simulink library "Hquad_control_LIB_LQR"  (Simulink 7.6)
settings: Solver=ode45  StartTime=0.0  StopTime=10.0  RelTol=1e-3
values from neighbouring files (symbols this model uses):
  g = 9.8065    [kostas_malakies.mat]    (also in kostas_malakies2.mat; load_PMModel.m = 9.81; main.m; main_last.m)
  K_lqr_x = [-0.863276621575 -0.709547355686 0.590253339062]    [kostas_malakies.mat]    (also in kostas_malakies2.mat)
  K_lqr_y = [0.862865129123 0.706975959941 0.571517383363]    [kostas_malakies.mat]    (also in kostas_malakies2.mat)
  K_lqr_yaw = [2.45277664624 0.892670523904]    [kostas_malakies.mat]    (also in kostas_malakies2.mat)
  K_lqr_z = [-2.51059156801 -2.42233318314]    [kostas_malakies.mat]    (also in kostas_malakies2.mat)
  mass = 0.66    [kostas_malakies.mat]    (also in kostas_malakies2.mat; load_PMModel.m = 0.687; main_last.m)
  MAX_ANGLE = 0.261799387799    [kostas_malakies.mat]    (also in kostas_malakies2.mat; main.m; main_last.m)
  MAX_FORCE = 2    [kostas_malakies.mat]    (also in kostas_malakies2.mat; main.m; main_last.m)
  MAX_YAW_RATE = 3.14159265359    [kostas_malakies.mat]    (also in kostas_malakies2.mat; main.m; main_last.m)
  traj_FG =     [kostas.mat]    (also in kostas_malakies.mat; kostas_malakies2.mat; main_last.m = ReferenceCreator(maxdisty,maxdistz,scale_y,scale_z); traj_helix.mat)
libraries: Hquad_control_LIB_LQR x13, simulink x9, Hquad_control_LIB_MPC x8
settings Model: Creator=andi  LastModifiedBy=burrimi

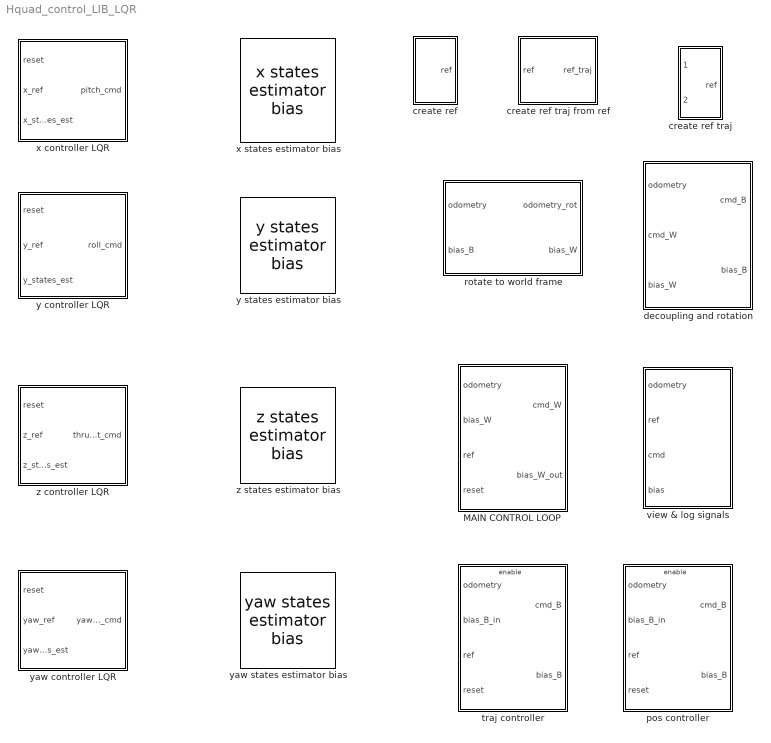
== system Hquad_control_LIB_LQR ==
  MAIN CONTROL LOOP : Subsystem  Priority=2  TreatAsAtomicUnit=on
  create ref : Subsystem
  create ref traj : Subsystem
  create ref traj from ref : Subsystem
  decoupling and rotation : Subsystem  Priority=3  TreatAsAtomicUnit=on
  pos controller : Subsystem
  rotate to world frame : Subsystem  Priority=1
  traj controller : Subsystem
  view & log signals : Subsystem
  "x controller LQR  " : Subsystem
  x states estimator bias : Hquad_control_LIB_MPC/x states estimator bias  SystemSampleTime=-1
  y controller LQR : Subsystem
  y states estimator bias : Hquad_control_LIB_MPC/y states estimator bias  SystemSampleTime=-1
  yaw controller LQR : Subsystem
  yaw states estimator bias : Hquad_control_LIB_MPC/yaw states estimator bias  SystemSampleTime=-1
  z controller LQR : Subsystem
  z states estimator bias : Hquad_control_LIB_MPC/z states estimator bias  SystemSampleTime=-1

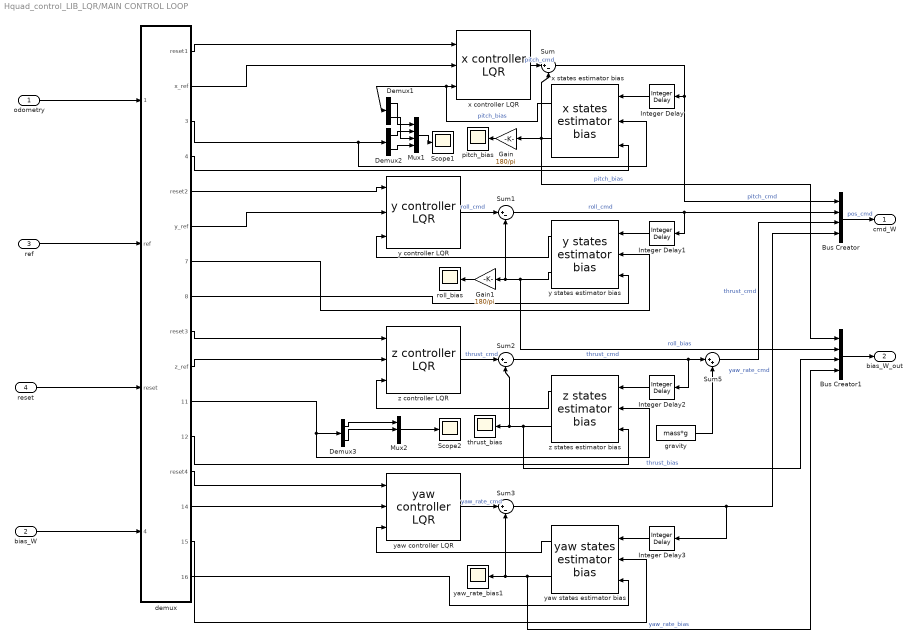
== system Hquad_control_LIB_LQR/MAIN CONTROL LOOP ==
  odometry : Inport
  bias_W : Inport  Port=2
  ref : Inport  Port=3
  reset : Inport  Port=4
  Bus Creator : BusCreator
  Bus Creator1 : BusCreator
  Demux1 : Demux  Outputs=3
  Demux2 : Demux  Outputs=3
  Demux3 : Demux  Outputs=2
  Gain : Gain  Gain=180/pi
  Gain1 : Gain  Gain=180/pi
  Integer Delay{,1..3} (4 alike) : simulink/Discrete/Integer Delay  NumDelays=1  vinit=0.0  samptime=-1
  Mux1 : Mux
  Mux2 : Mux  Inputs=5
  Scope1 : Scope
      settings: YMin=-0.05  YMax=1.05  SaveName=ScopeData6
  Scope2 : Scope
      settings: YMin=-0.4  YMax=1.4  SaveName=ScopeData15
  Sum{,1..3} (4 alike) : Sum  Inputs=|+-
  Sum5 : Sum  Inputs=|++
  demux : Subsystem
  gravity : Constant  Value=mass*g
  pitch_bias : Scope
      settings: YMin=0  YMax=3.75  SaveName=ScopeData7
  roll_bias : Scope
      settings: YMin=-1  YMax=1  SaveName=ScopeData12
  thrust_bias : Scope
      settings: YMin=0  YMax=0.3  SaveName=ScopeData13
  "x controller LQR  " : Hquad_control_LIB_LQR/x controller LQR    SystemSampleTime=-1
  x states estimator bias : Hquad_control_LIB_MPC/x states estimator bias  SystemSampleTime=-1
  y controller LQR : Hquad_control_LIB_LQR/y controller LQR  SystemSampleTime=-1
  y states estimator bias : Hquad_control_LIB_MPC/y states estimator bias  SystemSampleTime=-1
  yaw controller LQR : Hquad_control_LIB_LQR/yaw controller LQR  SystemSampleTime=-1
  yaw states estimator bias : Hquad_control_LIB_MPC/yaw states estimator bias  SystemSampleTime=-1
  yaw_rate_bias1 : Scope
      settings: YMin=-1  YMax=1  SaveName=ScopeData16
  z controller LQR : Hquad_control_LIB_LQR/z controller LQR  SystemSampleTime=-1
  z states estimator bias : Hquad_control_LIB_MPC/z states estimator bias  SystemSampleTime=-1
  cmd_W : Outport
  bias_W_out : Outport  Port=2
  wires:
  x states estimator bias/1 -> Demux1/1, "x controller LQR  "/3  "pitch_bias"
  demux/14(yaw_ref) -> yaw controller LQR/2
  demux/11(z_states_meas) -> Demux3/1, z states estimator bias/2
  demux/7(y_states_meas) -> y states estimator bias/2
  demux/3(x_states_meas) -> Demux2/1, x states estimator bias/2
  Bus Creator/1 -> cmd_W/1  "pos_cmd"
  demux/13(reset4) -> yaw controller LQR/1
  demux/9(reset3) -> z controller LQR/1
  demux/6(y_ref) -> y controller LQR/2
  demux/5(reset2) -> y controller LQR/1
  demux/1(reset1) -> "x controller LQR  "/1
  reset/1 -> demux/3(reset)
  ref/1 -> demux/2(ref)
  odometry/1 -> demux/1(odometry)
  Integer Delay2/1 -> z states estimator bias/1
  Integer Delay1/1 -> y states estimator bias/1
  demux/2(x_ref) -> "x controller LQR  "/2
  demux/10(z_ref) -> z controller LQR/2
  z states estimator bias/1 -> z controller LQR/3
  Mux2/1 -> Scope2/1
  Demux3/1 -> Mux2/1
  Demux3/2 -> Mux2/3
  Integer Delay/1 -> x states estimator bias/1
  y states estimator bias/1 -> y controller LQR/3
  Demux1/1 -> Mux1/1
  Demux2/1 -> Mux1/2
  Mux1/1 -> Scope1/1
  "x controller LQR  "/1 -> Sum/1  "pitch_cmd"
  Sum/1 -> Integer Delay/1, Bus Creator/1  "pitch_cmd"
  y controller LQR/1 -> Sum1/1  "roll_cmd"
  Sum1/1 -> Integer Delay1/1, Bus Creator/2  "roll_cmd"
  y states estimator bias/2 -> Gain1/1, Sum1/2, Bus Creator1/2  "roll_bias"
  z states estimator bias/2 -> Bus Creator1/3, thrust_bias/1, Sum2/2  "thrust_bias"
  z controller LQR/1 -> Sum2/1  "thrust_cmd"
  Sum2/1 -> Integer Delay2/1, Sum5/1  "thrust_cmd"
  Bus Creator1/1 -> bias_W_out/1
  gravity/1 -> Sum5/2
  Sum5/1 -> Bus Creator/3  "thrust_cmd"
  Gain/1 -> pitch_bias/1
  Gain1/1 -> roll_bias/1
  demux/15(yaw_states_meas) -> yaw states estimator bias/2
  Demux1/3 -> Mux1/3
  Demux2/3 -> Mux1/4
  x states estimator bias/2 -> Gain/1, Bus Creator1/1, Sum/2  "pitch_bias"
  Integer Delay3/1 -> yaw states estimator bias/1
  yaw states estimator bias/1 -> yaw controller LQR/3
  yaw states estimator bias/2 -> yaw_rate_bias1/1, Sum3/2, Bus Creator1/4  "yaw_rate_bias"
  yaw controller LQR/1 -> Sum3/1  "yaw_rate_cmd"
  Sum3/1 -> Bus Creator/4, Integer Delay3/1  "yaw_rate_cmd"
  bias_W/1 -> demux/4(bias_W)
  demux/16(yaw_rate_bias) -> yaw states estimator bias/3
  demux/12(thrust_bias) -> z states estimator bias/3
  demux/8(roll_bias) -> y states estimator bias/3
  demux/4(pitch_bias) -> x states estimator bias/3

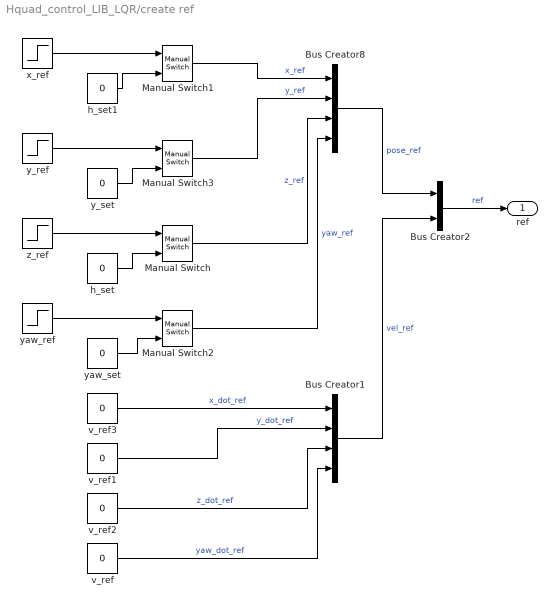
== system Hquad_control_LIB_LQR/create ref ==
  Bus Creator1 : BusCreator
  Bus Creator2 : BusCreator  Inputs=2
  Bus Creator8 : BusCreator
  Manual Switch{,1..3} (4 alike) : simulink/Signal Routing/Manual Switch  SystemSampleTime=-1  sw=1  action=0  varsize=off
  h_set : Constant  Value=0  OutDataTypeStr=double  SampleTime=-1
  h_set1 : Constant  Value=0  OutDataTypeStr=double  SampleTime=-1
  v_ref{,1..3} (4 alike) : Constant  Value=0  OutDataTypeStr=double  SampleTime=-1
  x_ref : Step  Time=5  SampleTime=0
  y_ref : Step  Time=15  SampleTime=0
  y_set : Constant  Value=0  OutDataTypeStr=double  SampleTime=-1
  yaw_ref : Step  Time=20  After=pi  SampleTime=0
  "yaw_set  " : Constant  Value=0  OutDataTypeStr=double  SampleTime=-1
  z_ref : Step  Time=15  SampleTime=0
  ref : Outport
  wires:
  yaw_ref/1 -> Manual Switch2/1
  "yaw_set  "/1 -> Manual Switch2/2
  h_set/1 -> Manual Switch/2
  z_ref/1 -> Manual Switch/1
  y_ref/1 -> Manual Switch3/1
  y_set/1 -> Manual Switch3/2
  h_set1/1 -> Manual Switch1/2
  Bus Creator2/1 -> ref/1  "ref"
  Bus Creator8/1 -> Bus Creator2/1  "pose_ref"
  Bus Creator1/1 -> Bus Creator2/2  "vel_ref"
  Manual Switch1/1 -> Bus Creator8/1  "x_ref"
  Manual Switch3/1 -> Bus Creator8/2  "y_ref"
  Manual Switch2/1 -> Bus Creator8/4  "yaw_ref"
  Manual Switch/1 -> Bus Creator8/3  "z_ref"
  v_ref/1 -> Bus Creator1/4  "yaw_dot_ref"
  v_ref3/1 -> Bus Creator1/1  "x_dot_ref"
  v_ref1/1 -> Bus Creator1/2  "y_dot_ref"
  v_ref2/1 -> Bus Creator1/3  "z_dot_ref"
  x_ref/1 -> Manual Switch1/1

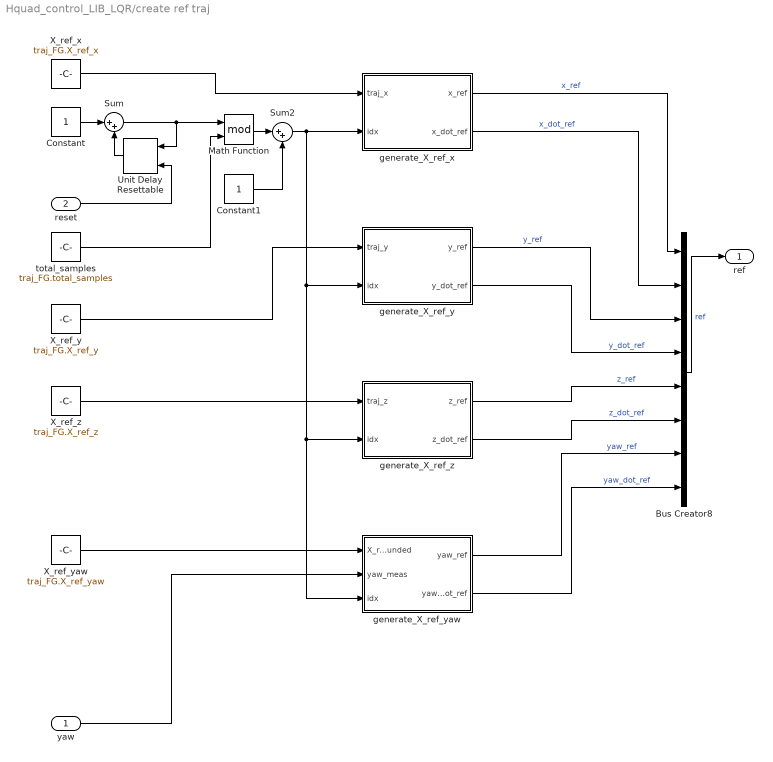
== system Hquad_control_LIB_LQR/create ref traj ==
  yaw : Inport
  reset : Inport  Port=2
  Bus Creator8 : BusCreator  Inputs=8
  Constant : Constant
  Constant1 : Constant
  Math Function : Math  Operator=mod  SaturateOnIntegerOverflow=on
  Sum : Sum  Inputs=|++
  Sum2 : Sum  Inputs=|++
  Unit Delay Resettable : simulink/Additional Math & Discrete/Additional Discrete/Unit Delay Resettable  SystemSampleTime=-1  vinit=0.0  tsamp=-1
  X_ref_x : Constant  Value=traj_FG.X_ref_x
  X_ref_y : Constant  Value=traj_FG.X_ref_y
  X_ref_yaw : Constant  Value=traj_FG.X_ref_yaw
  X_ref_z : Constant  Value=traj_FG.X_ref_z
  generate_X_ref_x : Stateflow chart  TreatAsAtomicUnit=on
  generate_X_ref_y : Stateflow chart  TreatAsAtomicUnit=on
  generate_X_ref_yaw : Stateflow chart  TreatAsAtomicUnit=on
  generate_X_ref_z : Stateflow chart  TreatAsAtomicUnit=on
  total_samples : Constant  Value=traj_FG.total_samples
  ref : Outport
  wires:
  reset/1 -> Unit Delay Resettable/2
  Bus Creator8/1 -> ref/1  "ref"
  Constant/1 -> Sum/1
  Unit Delay Resettable/1 -> Sum/2
  Sum/1 -> Unit Delay Resettable/1, Math Function/1
  total_samples/1 -> Math Function/2
  Math Function/1 -> Sum2/1
  X_ref_yaw/1 -> generate_X_ref_yaw/1(X_ref_yaw_unbounded)
  Constant1/1 -> Sum2/2
  yaw/1 -> generate_X_ref_yaw/2(yaw_meas)
  Sum2/1 -> generate_X_ref_x/2(idx), generate_X_ref_yaw/3(idx), generate_X_ref_z/2(idx), generate_X_ref_y/2(idx)
  X_ref_z/1 -> generate_X_ref_z/1(traj_z)
  X_ref_y/1 -> generate_X_ref_y/1(traj_y)
  X_ref_x/1 -> generate_X_ref_x/1(traj_x)
  generate_X_ref_yaw/2(yaw_dot_ref) -> Bus Creator8/8  "yaw_dot_ref"
  generate_X_ref_yaw/1(yaw_ref) -> Bus Creator8/7  "yaw_ref"
  generate_X_ref_z/2(z_dot_ref) -> Bus Creator8/6  "z_dot_ref"
  generate_X_ref_z/1(z_ref) -> Bus Creator8/5  "z_ref"
  generate_X_ref_y/2(y_dot_ref) -> Bus Creator8/4  "y_dot_ref"
  generate_X_ref_y/1(y_ref) -> Bus Creator8/3  "y_ref"
  generate_X_ref_x/2(x_dot_ref) -> Bus Creator8/2  "x_dot_ref"
  generate_X_ref_x/1(x_ref) -> Bus Creator8/1  "x_ref"

== system Hquad_control_LIB_LQR/create ref traj from ref ==
  ref : Inport
  Bus Creator8 : BusCreator
  Bus Selector1 : BusSelector  OutputSignals=pose_ref.x_ref,vel_ref.x_dot_ref,pose_ref.y_ref,vel_ref.y_dot_ref,pose_ref.z_ref,vel_ref.z_dot_ref,pose_ref.yaw_ref,vel_ref.yaw_dot_ref
  generate_X_ref_x : Stateflow chart  TreatAsAtomicUnit=on
  generate_X_ref_y : Stateflow chart  TreatAsAtomicUnit=on
  generate_X_ref_yaw : Stateflow chart  TreatAsAtomicUnit=on
  generate_X_ref_z : Stateflow chart  TreatAsAtomicUnit=on
  ref_traj : Outport
  wires:
  Bus Creator8/1 -> ref_traj/1  "ref"
  generate_X_ref_x/1(X_ref) -> Bus Creator8/1  "X_ref_x"
  generate_X_ref_y/1(X_ref) -> Bus Creator8/2  "X_ref_y"
  generate_X_ref_z/1(X_ref) -> Bus Creator8/3  "X_ref_z"
  generate_X_ref_yaw/1(X_ref) -> Bus Creator8/4  "X_ref_yaw"
  ref/1 -> Bus Selector1/1
  Bus Selector1/1 -> generate_X_ref_x/1(x_ref)  "<x_ref>"
  Bus Selector1/2 -> generate_X_ref_x/2(x_dot_ref)  "<x_dot_ref>"
  Bus Selector1/3 -> generate_X_ref_y/1(x_ref)  "<y_ref>"
  Bus Selector1/4 -> generate_X_ref_y/2(x_dot_ref)  "<y_dot_ref>"
  Bus Selector1/5 -> generate_X_ref_z/1(x_ref)  "<z_ref>"
  Bus Selector1/6 -> generate_X_ref_z/2(x_dot_ref)  "<z_dot_ref>"
  Bus Selector1/7 -> generate_X_ref_yaw/1(x_ref)  "<yaw_ref>"
  Bus Selector1/8 -> generate_X_ref_yaw/2(x_dot_ref)  "<yaw_dot_ref>"

== system Hquad_control_LIB_LQR/decoupling and rotation ==
  note: 
  odometry : Inport
  cmd_W : Inport  Port=2
  bias_W : Inport  Port=3
  Bus Selector1 : BusSelector  OutputSignals=rpy.yaw
  Bus Selector2 : BusSelector  OutputSignals=rpy.roll,rpy.pitch
  "decoupling " : Subsystem
  rotate_to_quat_frame : Subsystem
  cmd_B : Outport
  bias_B : Outport  Port=2
  wires:
  rotate_to_quat_frame/1("cmd_rot  ") -> cmd_B/1  "roll_cmd"
  "decoupling "/1("cmd_comp  ") -> rotate_to_quat_frame/2(cmd_comp)  "thrust_cmd"
  odometry/1 -> Bus Selector1/1, Bus Selector2/1
  Bus Selector1/1 -> rotate_to_quat_frame/1(yaw_meas)  "<yaw>"
  rotate_to_quat_frame/2(bias_rot) -> bias_B/1
  bias_W/1 -> rotate_to_quat_frame/3(bias)
  cmd_W/1 -> "decoupling "/3(cmd)
  Bus Selector2/1 -> "decoupling "/1("roll_meas  ")  "<roll>"
  Bus Selector2/2 -> "decoupling "/2("pitch_meas  ")  "<pitch>"

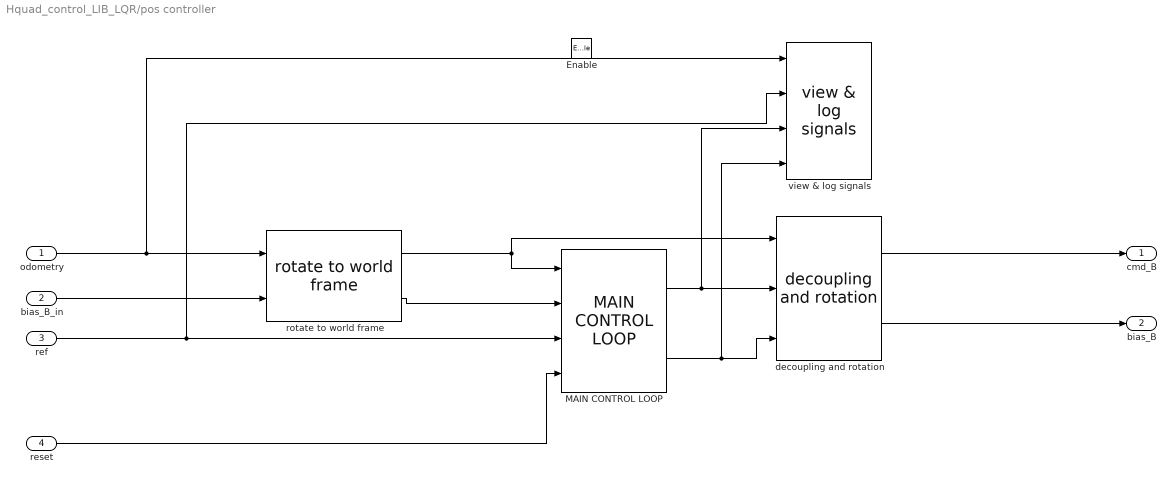
== system Hquad_control_LIB_LQR/pos controller ==
  odometry : Inport
  bias_B_in : Inport  Port=2
  ref : Inport  Port=3
  reset : Inport  Port=4
  Enable : EnablePort  StatesWhenEnabling=reset
  MAIN CONTROL LOOP : Hquad_control_LIB_LQR/MAIN CONTROL LOOP  Priority=2  SystemSampleTime=-1
  decoupling and rotation : Hquad_control_LIB_LQR/decoupling and rotation  Priority=3  SystemSampleTime=-1
  rotate to world frame : Hquad_control_LIB_LQR/rotate to world frame  Priority=1  SystemSampleTime=-1
  view & log signals : Hquad_control_LIB_LQR/view & log signals  SystemSampleTime=-1
  cmd_B : Outport
  bias_B : Outport  Port=2
  wires:
  MAIN CONTROL LOOP/1 -> view & log signals/3, decoupling and rotation/2
  odometry/1 -> view & log signals/1, rotate to world frame/1
  reset/1 -> MAIN CONTROL LOOP/4
  ref/1 -> view & log signals/2, MAIN CONTROL LOOP/3
  rotate to world frame/1 -> decoupling and rotation/1, MAIN CONTROL LOOP/1
  MAIN CONTROL LOOP/2 -> view & log signals/4, decoupling and rotation/3
  decoupling and rotation/1 -> cmd_B/1
  decoupling and rotation/2 -> bias_B/1
  rotate to world frame/2 -> MAIN CONTROL LOOP/2
  bias_B_in/1 -> rotate to world frame/2

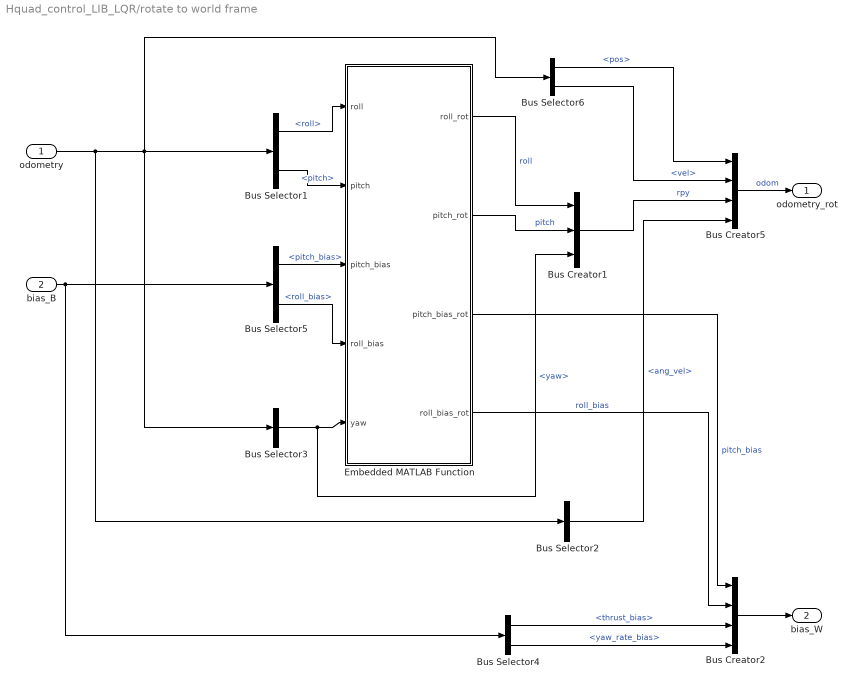
== system Hquad_control_LIB_LQR/rotate to world frame ==
  odometry : Inport
  bias_B : Inport  Port=2
  Bus Creator1 : BusCreator  Inputs=3
  Bus Creator2 : BusCreator
  Bus Creator5 : BusCreator
  Bus Selector1 : BusSelector  OutputSignals=rpy.roll,rpy.pitch
  Bus Selector2 : BusSelector  OutputSignals=ang_vel
  Bus Selector3 : BusSelector  OutputSignals=rpy.yaw
  Bus Selector4 : BusSelector  OutputSignals=thrust_bias,yaw_rate_bias
  Bus Selector5 : BusSelector  OutputSignals=pitch_bias,roll_bias
  Bus Selector6 : BusSelector  OutputSignals=pos,vel
  Embedded MATLAB Function : Stateflow chart  TreatAsAtomicUnit=on
  odometry_rot : Outport
  bias_W : Outport  Port=2
  wires:
  Bus Selector6/2 -> Bus Creator5/2  "<vel>"
  Bus Selector6/1 -> Bus Creator5/1  "<pos>"
  Bus Creator5/1 -> odometry_rot/1  "odom"
  Bus Selector3/1 -> Embedded MATLAB Function/5(yaw), Bus Creator1/3  "<yaw>"
  odometry/1 -> Bus Selector3/1, Bus Selector1/1, Bus Selector6/1, Bus Selector2/1
  Bus Selector2/1 -> Bus Creator5/4  "<ang_vel>"
  Bus Creator1/1 -> Bus Creator5/3  "rpy"
  Embedded MATLAB Function/1(roll_rot) -> Bus Creator1/1  "roll"
  Embedded MATLAB Function/2(pitch_rot) -> Bus Creator1/2  "pitch"
  Bus Selector1/1 -> Embedded MATLAB Function/1(roll)  "<roll>"
  Bus Selector1/2 -> Embedded MATLAB Function/2(pitch)  "<pitch>"
  Bus Creator2/1 -> bias_W/1
  Bus Selector4/2 -> Bus Creator2/4  "<yaw_rate_bias>"
  Bus Selector4/1 -> Bus Creator2/3  "<thrust_bias>"
  Bus Selector5/1 -> Embedded MATLAB Function/3(pitch_bias)  "<pitch_bias>"
  Bus Selector5/2 -> Embedded MATLAB Function/4(roll_bias)  "<roll_bias>"
  bias_B/1 -> Bus Selector5/1, Bus Selector4/1
  Embedded MATLAB Function/3(pitch_bias_rot) -> Bus Creator2/1  "pitch_bias"
  Embedded MATLAB Function/4(roll_bias_rot) -> Bus Creator2/2  "roll_bias"

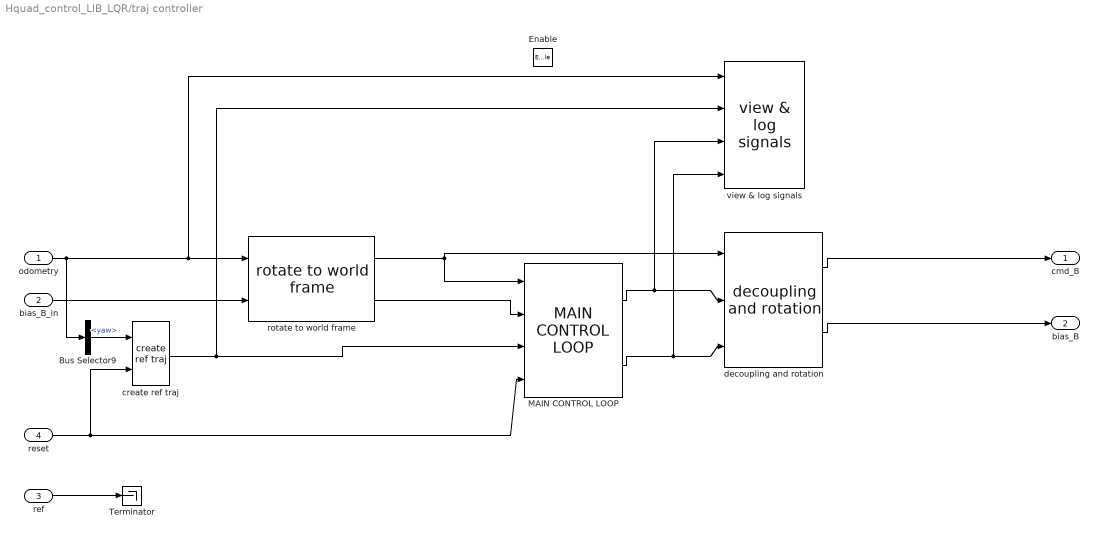
== system Hquad_control_LIB_LQR/traj controller ==
  odometry : Inport
  bias_B_in : Inport  Port=2
  ref : Inport  Port=3
  reset : Inport  Port=4
  Enable : EnablePort  StatesWhenEnabling=reset
  Bus Selector9 : BusSelector  OutputSignals=rpy.yaw
  MAIN CONTROL LOOP : Hquad_control_LIB_LQR/MAIN CONTROL LOOP  Priority=2  SystemSampleTime=-1
  Terminator : Terminator
  create ref traj : Hquad_control_LIB_LQR/create ref traj  SystemSampleTime=-1
  decoupling and rotation : Hquad_control_LIB_LQR/decoupling and rotation  Priority=3  SystemSampleTime=-1
  rotate to world frame : Hquad_control_LIB_LQR/rotate to world frame  Priority=1  SystemSampleTime=-1
  view & log signals : Hquad_control_LIB_LQR/view & log signals  SystemSampleTime=-1
  cmd_B : Outport
  bias_B : Outport  Port=2
  wires:
  ref/1 -> Terminator/1
  Bus Selector9/1 -> create ref traj/1  "<yaw>"
  bias_B_in/1 -> rotate to world frame/2
  rotate to world frame/2 -> MAIN CONTROL LOOP/2
  decoupling and rotation/2 -> bias_B/1
  decoupling and rotation/1 -> cmd_B/1
  MAIN CONTROL LOOP/2 -> decoupling and rotation/3, view & log signals/4
  reset/1 -> create ref traj/2, MAIN CONTROL LOOP/4
  odometry/1 -> Bus Selector9/1, rotate to world frame/1, view & log signals/1
  MAIN CONTROL LOOP/1 -> decoupling and rotation/2, view & log signals/3
  rotate to world frame/1 -> MAIN CONTROL LOOP/1, decoupling and rotation/1
  create ref traj/1 -> MAIN CONTROL LOOP/3, view & log signals/2

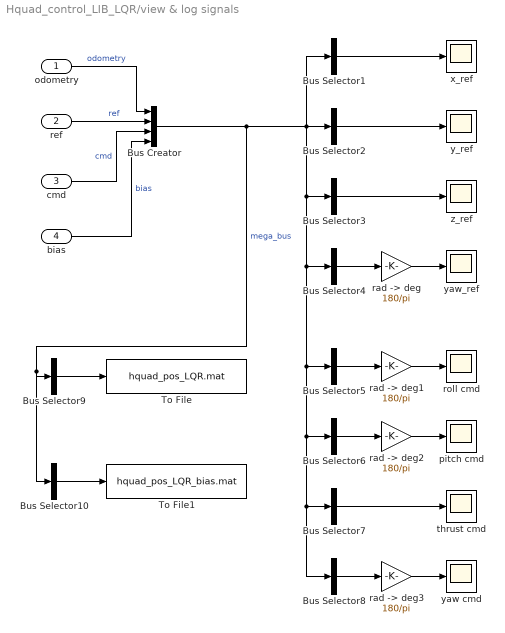
== system Hquad_control_LIB_LQR/view & log signals ==
  odometry : Inport
  ref : Inport  Port=2
  cmd : Inport  Port=3
  bias : Inport  Port=4
  Bus Creator : BusCreator
  Bus Selector1 : BusSelector  OutputSignals=odometry.pos.x,odometry.vel.x_dot,ref.pose_ref.x_ref,ref.vel_ref.x_dot_ref  OutputAsBus=on
  Bus Selector10 : BusSelector  OutputSignals=bias.pitch_bias,bias.roll_bias,bias.thrust_bias,bias.yaw_rate_bias  OutputAsBus=on
  Bus Selector2 : BusSelector  OutputSignals=odometry.pos.y,odometry.vel.y_dot,ref.pose_ref.y_ref,ref.vel_ref.y_dot_ref  OutputAsBus=on
  Bus Selector3 : BusSelector  OutputSignals=odometry.pos.z,odometry.vel.z_dot,ref.pose_ref.z_ref,ref.vel_ref.z_dot_ref  OutputAsBus=on
  Bus Selector4 : BusSelector  OutputSignals=odometry.rpy.yaw,odometry.ang_vel.ang_vel_z,ref.pose_ref.yaw_ref,ref.vel_ref.yaw_dot_ref  OutputAsBus=on
  Bus Selector5 : BusSelector  OutputSignals=odometry.rpy.roll,odometry.ang_vel.ang_vel_x,cmd.roll_cmd  OutputAsBus=on
  Bus Selector6 : BusSelector  OutputSignals=odometry.rpy.pitch,odometry.ang_vel.ang_vel_y,cmd.pitch_cmd  OutputAsBus=on
  Bus Selector7 : BusSelector  OutputSignals=odometry.pos.z,ref.pose_ref.z_ref,cmd.thrust_cmd  OutputAsBus=on
  Bus Selector8 : BusSelector  OutputSignals=odometry.rpy.yaw,odometry.ang_vel.ang_vel_z,cmd.yaw_rate_cmd  OutputAsBus=on
  Bus Selector9 : BusSelector  OutputSignals=odometry.pos.x,odometry.vel.x_dot,odometry.rpy.pitch,ref.pose_ref.x_ref,cmd.pitch_cmd,odometry.pos.y,odometry.vel.y_dot,odometry.rpy.roll,ref.pose_ref.y_ref,cmd.roll_cmd,odometry.pos.z,odometry.vel.z_dot,ref.pose_ref.z_ref,cmd.thrust_cmd,odometry.rpy.yaw,odometry.ang_vel.ang_vel_z,ref.pose_ref.yaw_ref,cmd.yaw_rate_cmd  OutputAsBus=on
  To File : ToFile  Filename=hquad_pos_LQR.mat  MatrixName=hquad_pos_LQR
  To File1 : ToFile  Filename=hquad_pos_LQR_bias.mat  MatrixName=hquad_pos_LQR_bias
  pitch cmd : Scope
      settings: YMin=-15  YMax=15  SaveName=ScopeData2
  rad -> deg{,1..3} (4 alike) : Gain  Gain=180/pi
  roll cmd : Scope
      settings: YMin=-100  YMax=100
  thrust cmd : Scope
      settings: YMin=-3  YMax=3  SaveName=ScopeData11
  x_ref : Scope
      settings: TimeRange=40  YMin=-1.5  YMax=1.5  SaveName=ScopeData3
  y_ref : Scope
      settings: TimeRange=40  YMin=-0.75  YMax=2.75
  yaw cmd : Scope
      settings: YMin=-60  YMax=-0  SaveName=ScopeData10
  yaw_ref : Scope
      settings: TimeRange=39.996  YMin=-1.5  YMax=8.5  SaveName=ScopeData8
  z_ref : Scope
      settings: TimeRange=40  YMin=-21  YMax=1  SaveName=ScopeData5
  wires:
  Bus Selector9/1 -> To File/1
  "rad -> deg"/1 -> yaw_ref/1
  "rad -> deg1"/1 -> roll cmd/1
  "rad -> deg2"/1 -> pitch cmd/1
  "rad -> deg3"/1 -> yaw cmd/1
  odometry/1 -> Bus Creator/1  "odometry"
  ref/1 -> Bus Creator/2  "ref"
  cmd/1 -> Bus Creator/3  "cmd"
  Bus Creator/1 -> Bus Selector1/1, Bus Selector2/1, Bus Selector3/1, Bus Selector4/1, Bus Selector5/1, Bus Selector6/1, Bus Selector7/1, Bus Selector8/1, Bus Selector9/1, Bus Selector10/1  "mega_bus"
  Bus Selector1/1 -> x_ref/1
  Bus Selector2/1 -> y_ref/1
  Bus Selector3/1 -> z_ref/1
  Bus Selector4/1 -> "rad -> deg"/1
  Bus Selector7/1 -> thrust cmd/1
  Bus Selector5/1 -> "rad -> deg1"/1
  Bus Selector6/1 -> "rad -> deg2"/1
  Bus Selector8/1 -> "rad -> deg3"/1
  bias/1 -> Bus Creator/4  "bias"
  Bus Selector10/1 -> To File1/1

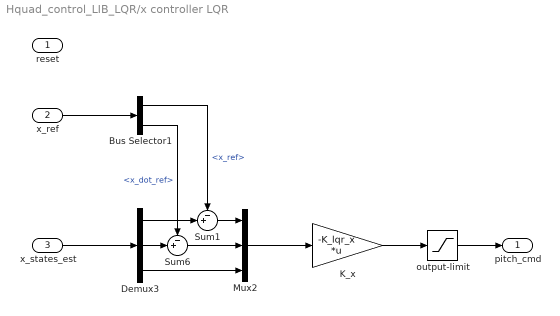
== system Hquad_control_LIB_LQR/x controller LQR   ==
  reset : Inport  PortDimensions=1
  "x_ref  " : Inport  Port=2  PortDimensions=2
  "x_states_est  " : Inport  Port=3
  Bus Selector1 : BusSelector  OutputSignals=x_ref,x_dot_ref
  Demux3 : Demux  Outputs=3
  K_x : Gain  Gain=-K_lqr_x  Multiplication=Matrix(K*u)
  Mux2 : Mux  Inputs=3
  Sum1 : Sum  Inputs=-+|
  Sum6 : Sum  Inputs=-+|
  output-limit : Saturate  UpperLimit=MAX_ANGLE  LowerLimit=-MAX_ANGLE
  "pitch_cmd   " : Outport  PortDimensions=1
  wires:
  Demux3/3 -> Mux2/3
  Demux3/2 -> Sum6/2
  Bus Selector1/2 -> Sum6/1  "<x_dot_ref>"
  Bus Selector1/1 -> Sum1/1  "<x_ref>"
  Sum6/1 -> Mux2/2
  "x_ref  "/1 -> Bus Selector1/1
  K_x/1 -> output-limit/1
  output-limit/1 -> "pitch_cmd   "/1
  "x_states_est  "/1 -> Demux3/1
  Mux2/1 -> K_x/1
  Demux3/1 -> Sum1/2
  Sum1/1 -> Mux2/1

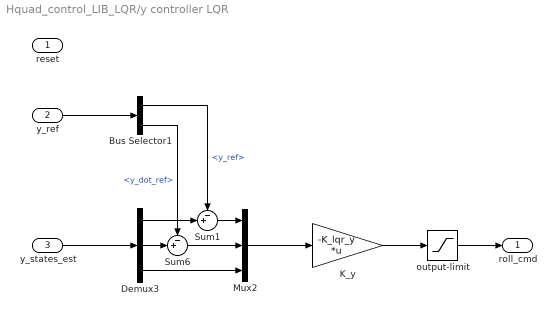
== system Hquad_control_LIB_LQR/y controller LQR ==
  reset : Inport  PortDimensions=1
  "y_ref " : Inport  Port=2  PortDimensions=2
  y_states_est : Inport  Port=3
  Bus Selector1 : BusSelector  OutputSignals=y_ref,y_dot_ref
  Demux3 : Demux  Outputs=3
  K_y : Gain  Gain=-K_lqr_y  Multiplication=Matrix(K*u)
  Mux2 : Mux  Inputs=3
  Sum1 : Sum  Inputs=-+|
  Sum6 : Sum  Inputs=-+|
  output-limit : Saturate  UpperLimit=MAX_ANGLE  LowerLimit=-MAX_ANGLE
  "roll_cmd   " : Outport  PortDimensions=1
  wires:
  Demux3/3 -> Mux2/3
  Demux3/2 -> Sum6/2
  Bus Selector1/2 -> Sum6/1  "<y_dot_ref>"
  Bus Selector1/1 -> Sum1/1  "<y_ref>"
  Sum6/1 -> Mux2/2
  "y_ref "/1 -> Bus Selector1/1
  K_y/1 -> output-limit/1
  output-limit/1 -> "roll_cmd   "/1
  y_states_est/1 -> Demux3/1
  Mux2/1 -> K_y/1
  Demux3/1 -> Sum1/2
  Sum1/1 -> Mux2/1

== system Hquad_control_LIB_LQR/yaw controller LQR ==
  reset : Inport  PortDimensions=1
  "yaw_ref " : Inport  Port=2  PortDimensions=2
  yaw_states_est : Inport  Port=3
  Bus Selector1 : BusSelector  OutputSignals=yaw_ref,yaw_dot_ref
  Demux3 : Demux  Outputs=2
  K_yaw : Gain  Gain=-K_lqr_yaw  Multiplication=Matrix(K*u)
  Mux2 : Mux  Inputs=2
  Sum1 : Sum  Inputs=-+|
  Sum6 : Sum  Inputs=-+|
  output-limit : Saturate  UpperLimit=MAX_YAW_RATE  LowerLimit=-MAX_YAW_RATE
  "yaw_rate_cmd " : Outport  PortDimensions=1
  wires:
  Demux3/2 -> Sum6/2
  Bus Selector1/2 -> Sum6/1  "<yaw_dot_ref>"
  Bus Selector1/1 -> Sum1/1  "<yaw_ref>"
  Sum6/1 -> Mux2/2
  "yaw_ref "/1 -> Bus Selector1/1
  K_yaw/1 -> output-limit/1
  output-limit/1 -> "yaw_rate_cmd "/1
  yaw_states_est/1 -> Demux3/1
  Mux2/1 -> K_yaw/1
  Demux3/1 -> Sum1/2
  Sum1/1 -> Mux2/1

== system Hquad_control_LIB_LQR/z controller LQR ==
  reset : Inport  PortDimensions=1
  "z_ref " : Inport  Port=2  PortDimensions=2
  z_states_est : Inport  Port=3
  Bus Selector1 : BusSelector  OutputSignals=z_ref,z_dot_ref
  Demux3 : Demux  Outputs=2
  K_z : Gain  Gain=-K_lqr_z  Multiplication=Matrix(K*u)
  Mux2 : Mux  Inputs=2
  Sum1 : Sum  Inputs=-+|
  Sum6 : Sum  Inputs=-+|
  output-limit : Saturate  UpperLimit=MAX_FORCE  LowerLimit=-MAX_FORCE
  "thrust_cmd   " : Outport  PortDimensions=1
  wires:
  Demux3/2 -> Sum6/2
  Bus Selector1/2 -> Sum6/1  "<z_dot_ref>"
  Bus Selector1/1 -> Sum1/1  "<z_ref>"
  Sum6/1 -> Mux2/2
  "z_ref "/1 -> Bus Selector1/1
  K_z/1 -> output-limit/1
  output-limit/1 -> "thrust_cmd   "/1
  z_states_est/1 -> Demux3/1
  Mux2/1 -> K_z/1
  Demux3/1 -> Sum1/2
  Sum1/1 -> Mux2/1

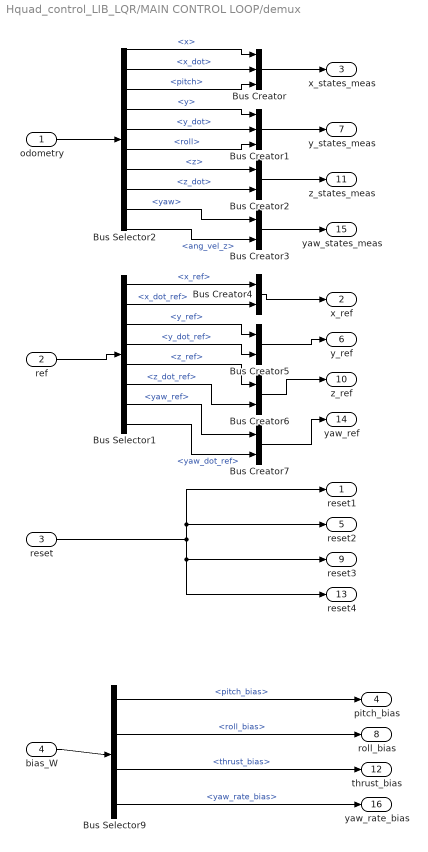
== system Hquad_control_LIB_LQR/MAIN CONTROL LOOP/demux ==
  odometry : Inport
  ref : Inport  Port=2
  reset : Inport  Port=3
  bias_W : Inport  Port=4
  Bus Creator : BusCreator  Inputs=3
  Bus Creator1 : BusCreator  Inputs=3
  Bus Creator{2..7} (6 alike) : BusCreator  Inputs=2
  Bus Selector1 : BusSelector  OutputSignals=pose_ref.x_ref,vel_ref.x_dot_ref,pose_ref.y_ref,vel_ref.y_dot_ref,pose_ref.z_ref,vel_ref.z_dot_ref,pose_ref.yaw_ref,vel_ref.yaw_dot_ref
  Bus Selector2 : BusSelector  OutputSignals=pos.x,vel.x_dot,rpy.pitch,pos.y,vel.y_dot,rpy.roll,pos.z,vel.z_dot,rpy.yaw,ang_vel.ang_vel_z
  Bus Selector9 : BusSelector  OutputSignals=pitch_bias,roll_bias,thrust_bias,yaw_rate_bias
  reset1 : Outport
  x_ref : Outport  Port=2
  x_states_meas : Outport  Port=3  PortDimensions=3
  pitch_bias : Outport  Port=4
  reset2 : Outport  Port=5
  y_ref : Outport  Port=6
  y_states_meas : Outport  Port=7  PortDimensions=3
  roll_bias : Outport  Port=8
  reset3 : Outport  Port=9
  z_ref : Outport  Port=10
  z_states_meas : Outport  Port=11  PortDimensions=2
  thrust_bias : Outport  Port=12
  reset4 : Outport  Port=13
  yaw_ref : Outport  Port=14
  yaw_states_meas : Outport  Port=15  PortDimensions=2
  yaw_rate_bias : Outport  Port=16
  wires:
  Bus Creator6/1 -> z_ref/1
  ref/1 -> Bus Selector1/1
  Bus Selector1/1 -> Bus Creator4/1  "<x_ref>"
  Bus Creator7/1 -> yaw_ref/1
  Bus Creator5/1 -> y_ref/1
  Bus Creator4/1 -> x_ref/1
  Bus Selector1/3 -> Bus Creator5/1  "<y_ref>"
  Bus Selector1/5 -> Bus Creator6/1  "<z_ref>"
  Bus Selector1/7 -> Bus Creator7/1  "<yaw_ref>"
  reset/1 -> reset1/1, reset2/1, reset4/1, reset3/1
  Bus Creator3/1 -> yaw_states_meas/1
  Bus Creator2/1 -> z_states_meas/1
  Bus Selector2/10 -> Bus Creator3/2  "<ang_vel_z>"
  Bus Selector2/9 -> Bus Creator3/1  "<yaw>"
  Bus Selector2/8 -> Bus Creator2/2  "<z_dot>"
  Bus Selector2/7 -> Bus Creator2/1  "<z>"
  Bus Creator1/1 -> y_states_meas/1
  Bus Selector2/5 -> Bus Creator1/2  "<y_dot>"
  Bus Selector2/4 -> Bus Creator1/1  "<y>"
  Bus Selector2/2 -> Bus Creator/2  "<x_dot>"
  Bus Selector2/1 -> Bus Creator/1  "<x>"
  Bus Creator/1 -> x_states_meas/1
  odometry/1 -> Bus Selector2/1
  Bus Selector2/3 -> Bus Creator/3  "<pitch>"
  Bus Selector2/6 -> Bus Creator1/3  "<roll>"
  bias_W/1 -> Bus Selector9/1
  Bus Selector9/1 -> pitch_bias/1  "<pitch_bias>"
  Bus Selector9/2 -> roll_bias/1  "<roll_bias>"
  Bus Selector9/3 -> thrust_bias/1  "<thrust_bias>"
  Bus Selector9/4 -> yaw_rate_bias/1  "<yaw_rate_bias>"
  Bus Selector1/2 -> Bus Creator4/2  "<x_dot_ref>"
  Bus Selector1/4 -> Bus Creator5/2  "<y_dot_ref>"
  Bus Selector1/6 -> Bus Creator6/2  "<z_dot_ref>"
  Bus Selector1/8 -> Bus Creator7/2  "<yaw_dot_ref>"

== system Hquad_control_LIB_LQR/decoupling and rotation/decoupling  ==
  "roll_meas  " : Inport  PortDimensions=1
  "pitch_meas  " : Inport  Port=2  PortDimensions=1
  cmd : Inport  Port=3
  Bus Creator : BusCreator
  Bus Selector3 : BusSelector  OutputSignals=pitch_cmd,roll_cmd,thrust_cmd,yaw_rate_cmd
  Embedded MATLAB Function : Stateflow chart  TreatAsAtomicUnit=on
  g : Constant  Value=g
  mass : Constant  Value=mass
  "cmd_comp  " : Outport
  wires:
  g/1 -> Embedded MATLAB Function/7(g)
  mass/1 -> Embedded MATLAB Function/6(m)
  Bus Selector3/3 -> Embedded MATLAB Function/5(thrust)  "<thrust_cmd>"
  Bus Selector3/2 -> Embedded MATLAB Function/4(roll_cmd)  "<roll_cmd>"
  Bus Selector3/1 -> Embedded MATLAB Function/3(pitch_cmd)  "<pitch_cmd>"
  Embedded MATLAB Function/1(pitch_cmd_comp) -> Bus Creator/1  "pitch_cmd"
  Embedded MATLAB Function/2(roll_cmd_comp) -> Bus Creator/2  "roll_cmd"
  Embedded MATLAB Function/3(thrust_comp) -> Bus Creator/3  "thrust_cmd"
  Bus Creator/1 -> "cmd_comp  "/1
  Bus Selector3/4 -> Bus Creator/4  "<yaw_rate_cmd>"
  cmd/1 -> Bus Selector3/1
  "pitch_meas  "/1 -> Embedded MATLAB Function/1(pitch_meas)
  "roll_meas  "/1 -> Embedded MATLAB Function/2(roll_meas)

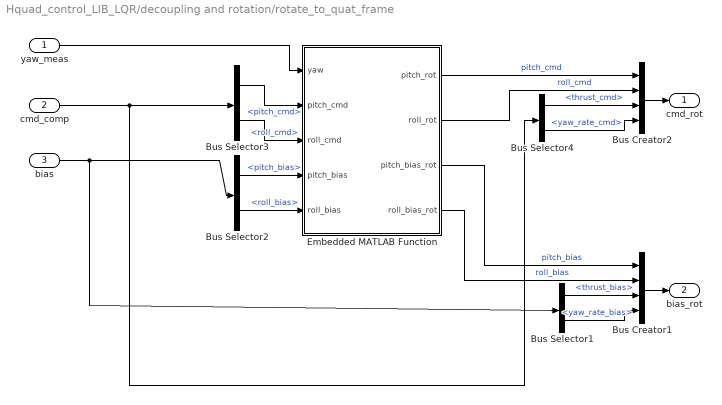
== system Hquad_control_LIB_LQR/decoupling and rotation/rotate_to_quat_frame ==
  yaw_meas : Inport
  cmd_comp : Inport  Port=2
  bias : Inport  Port=3
  Bus Creator1 : BusCreator
  Bus Creator2 : BusCreator
  Bus Selector1 : BusSelector  OutputSignals=thrust_bias,yaw_rate_bias
  Bus Selector2 : BusSelector  OutputSignals=pitch_bias,roll_bias
  Bus Selector3 : BusSelector  OutputSignals=pitch_cmd,roll_cmd
  Bus Selector4 : BusSelector  OutputSignals=thrust_cmd,yaw_rate_cmd
  Embedded MATLAB Function : Stateflow chart  TreatAsAtomicUnit=on
  "cmd_rot  " : Outport
  bias_rot : Outport  Port=2
  wires:
  Bus Selector1/2 -> Bus Creator1/4  "<yaw_rate_bias>"
  Bus Selector1/1 -> Bus Creator1/3  "<thrust_bias>"
  Bus Selector4/2 -> Bus Creator2/4  "<yaw_rate_cmd>"
  Bus Selector4/1 -> Bus Creator2/3  "<thrust_cmd>"
  Embedded MATLAB Function/2(roll_rot) -> Bus Creator2/2  "roll_cmd"
  Embedded MATLAB Function/1(pitch_rot) -> Bus Creator2/1  "pitch_cmd"
  cmd_comp/1 -> Bus Selector4/1, Bus Selector3/1
  Bus Selector3/1 -> Embedded MATLAB Function/2(pitch_cmd)  "<pitch_cmd>"
  Bus Selector3/2 -> Embedded MATLAB Function/3(roll_cmd)  "<roll_cmd>"
  Bus Creator2/1 -> "cmd_rot  "/1
  Embedded MATLAB Function/4(roll_bias_rot) -> Bus Creator1/2  "roll_bias"
  Embedded MATLAB Function/3(pitch_bias_rot) -> Bus Creator1/1  "pitch_bias"
  Bus Selector2/2 -> Embedded MATLAB Function/5(roll_bias)  "<roll_bias>"
  Bus Selector2/1 -> Embedded MATLAB Function/4(pitch_bias)  "<pitch_bias>"
  Bus Creator1/1 -> bias_rot/1
  bias/1 -> Bus Selector1/1, Bus Selector2/1
  yaw_meas/1 -> Embedded MATLAB Function/1(yaw)

== matlab function decoupling and rotation/decoupling /Embedded MATLAB Function ==
  data: pitch_cmd_comp output double; roll_cmd_comp output double; pitch_meas input double; thrust_comp output double; roll_meas input double; pitch_cmd input double; roll_cmd input double; thrust input double; m input double; g input double
function [pitch_cmd_comp, roll_cmd_comp, thrust_comp]  = fcn(pitch_meas, roll_meas, pitch_cmd, roll_cmd, thrust,m,g)
%#eml

thrust_comp=thrust/(cos(pitch_meas)*cos(roll_meas));

pitch_cmd_comp = m*g/thrust_comp*pitch_cmd;
roll_cmd_comp = m*g/thrust_comp*roll_cmd;

% pitch_cmd_comp=pitch_cmd;
% roll_cmd_comp=roll_cmd;
% pitch_cmd_comp = atan(Fx/(-thrust_comp));
% roll_cmd_comp = atan(Fy/(thrust_comp));

% pitch_cmd_comp = atan(-g*m*pitch_cmd/(-thrust));
% roll_cmd_comp = atan(g*m*roll_cmd*cos(pitch_meas)/(thrust));

== matlab function create ref traj/generate_X_ref_x ==
  data: traj_x input double; x_ref output double; idx input double; x_dot_ref output double
function [x_ref, x_dot_ref]  = fcn(traj_x,idx)


x_ref=traj_x(1,idx);
x_dot_ref=traj_x(2,idx);

== matlab function decoupling and rotation/rotate_to_quat_frame/Embedded MATLAB Function ==
  data: yaw input double; pitch_rot output double; pitch_cmd input double; roll_cmd input double; pitch_bias input double; roll_bias input double; roll_rot output double; pitch_bias_rot output double; roll_bias_rot output double
function [pitch_rot,roll_rot, pitch_bias_rot,roll_bias_rot] = fcn(yaw, pitch_cmd, roll_cmd, pitch_bias, roll_bias)

sin_yaw=sin(yaw);
cos_yaw=cos(yaw);

R=[cos_yaw, sin_yaw; -sin_yaw, cos_yaw];

temp=R'*[pitch_cmd;roll_cmd];
pitch_rot=temp(1);
roll_rot=temp(2);

temp=R'*[pitch_bias;roll_bias];
pitch_bias_rot=temp(1);
roll_bias_rot=temp(2);

== matlab function create ref traj from ref/generate_X_ref_x ==
  data: x_ref input double; x_dot_ref input double; X_ref output double
function X_ref  = fcn(x_ref, x_dot_ref)
   
pred_horizon=30;

X_ref_temp=[x_ref*ones(1,pred_horizon+1); x_dot_ref*ones(1,pred_horizon+1); zeros(1,pred_horizon+1)];

X_ref=reshape(X_ref_temp,1,[])';

== matlab function create ref traj from ref/generate_X_ref_y ==
  data: x_ref input double; x_dot_ref input double; X_ref output double
function X_ref  = fcn(x_ref, x_dot_ref)
   
pred_horizon=30;

X_ref_temp=[x_ref*ones(1,pred_horizon+1); x_dot_ref*ones(1,pred_horizon+1); zeros(1,pred_horizon+1)];

X_ref=reshape(X_ref_temp,1,[])';

== matlab function create ref traj from ref/generate_X_ref_yaw ==
  data: x_ref input double; x_dot_ref input double; X_ref output double
function X_ref  = fcn(x_ref, x_dot_ref)
   
pred_horizon=30;

X_ref_temp=[x_ref*ones(1,pred_horizon+1); x_dot_ref*ones(1,pred_horizon+1)];

X_ref=reshape(X_ref_temp,1,[])';

== matlab function create ref traj from ref/generate_X_ref_z ==
  data: x_ref input double; x_dot_ref input double; X_ref output double
function X_ref  = fcn(x_ref, x_dot_ref)
   
pred_horizon=30;

X_ref_temp=[x_ref*ones(1,pred_horizon+1); x_dot_ref*ones(1,pred_horizon+1)];

X_ref=reshape(X_ref_temp,1,[])';

== matlab function create ref traj/generate_X_ref_y ==
  data: traj_y input double; y_ref output double; idx input double; y_dot_ref output double
function [y_ref, y_dot_ref]  = fcn(traj_y,idx)


y_ref=traj_y(1,idx);
y_dot_ref=traj_y(2,idx);

== matlab function create ref traj/generate_X_ref_yaw ==
  data: X_ref_yaw_unbounded input double; yaw_ref output double; yaw_meas input double; idx input double; yaw_dot_ref output double
function [yaw_ref,yaw_dot_ref]  = fcn(X_ref_yaw_unbounded,yaw_meas,idx)


yaw0=X_ref_yaw_unbounded(1,idx);
yaw_diff=yaw_meas-yaw0;


yaw_offset=round(yaw_diff/(2*pi))*2*pi;


yaw_ref=X_ref_yaw_unbounded(1,idx)+yaw_offset;
yaw_dot_ref=X_ref_yaw_unbounded(2,idx);

== matlab function create ref traj/generate_X_ref_z ==
  data: traj_z input double; z_ref output double; idx input double; z_dot_ref output double
function [z_ref,z_dot_ref]  = fcn(traj_z,idx)

z_ref=traj_z(1,idx);
z_dot_ref=traj_z(2,idx);

== matlab function rotate to world frame/Embedded MATLAB Function ==
  data: roll input double; pitch input double; pitch_bias input double; roll_bias input double; roll_rot output double; yaw input double; pitch_rot output double; pitch_bias_rot output double; roll_bias_rot output double
function [roll_rot,pitch_rot,pitch_bias_rot,roll_bias_rot] = fcn(roll,pitch,pitch_bias,roll_bias,yaw)
%#eml


sin_yaw=sin(yaw);
cos_yaw=cos(yaw);

R=[cos_yaw, sin_yaw; -sin_yaw, cos_yaw];

temp=R*[pitch;roll];
pitch_rot=temp(1);
roll_rot=temp(2);

temp=R*[pitch_bias;roll_bias];
pitch_bias_rot=temp(1);
roll_bias_rot=temp(2);
